simulink model "sipo_4bit"  (R2025b)
settings: Solver=VariableStepAuto  StartTime=0.0  StopTime=10.0  RelTol=1e-3
libraries: simulink_extras x5
settings Model: Creator=Johan  LastModifiedBy=Johan

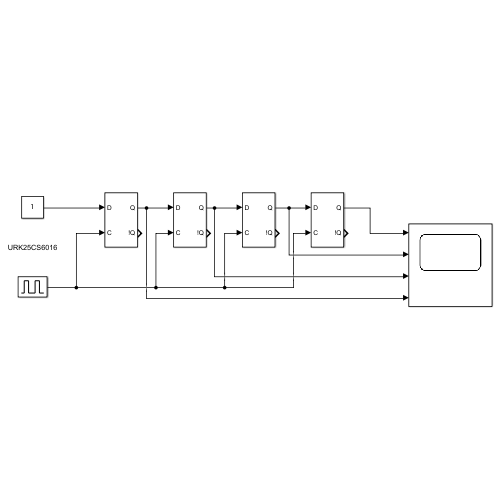
[thumbnail: Simulink's stored preview of the top-level diagram]
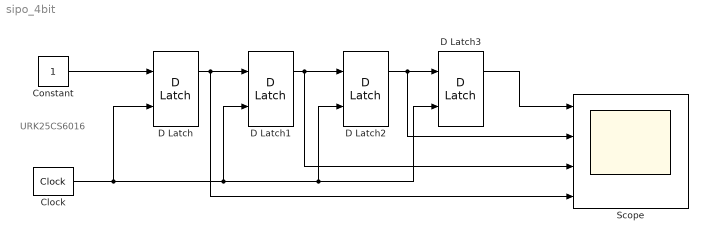
== system sipo_4bit ==
  note: URK25CS6016
  Clock : simulink_extras/Flip Flops/Clock  period=2
  Constant : Constant  OutDataTypeStr=boolean
  D Latch{,1..3} (4 alike) : simulink_extras/Flip Flops/D Latch
  Scope : Scope  NumInputPorts=4
      settings: ActiveDisplayYMinimum=0.9  ActiveDisplayYMaximum=1.1
  wires:
  Constant/1 -> D Latch/1
  Clock/1 -> D Latch1/2, D Latch2/2, D Latch3/2, D Latch/2
  D Latch/1 -> D Latch1/1, Scope/4
  D Latch1/1 -> D Latch2/1, Scope/3
  D Latch2/1 -> Scope/2, D Latch3/1
  D Latch3/1 -> Scope/1
